simulink model "control"  (R2023a)
settings: Solver=ode45  StartTime=0.0  StopTime=T  RelTol=1e-3
values from neighbouring files (symbols this model uses):
  z = ismembertol(env.V,[X(x,x),Y(y,y)], 'ByRows', true)    [Environment.m]
undefined symbols (not defined in the file or in its folder): hctrl, Tc
settings Model: Creator=Luca  LastModifiedBy=nick
settings SolverCC: AlgebraicLoopSolver=TrustRegion
settings DataIOCC: ReturnWorkspaceOutputs=off
settings DebuggingCC: UnconnectedInputMsg=warning  UnconnectedOutputMsg=warning  UnconnectedLineMsg=warning  ArithmeticOperatorsInVariantConditions=warning
settings ModelReferenceCC: EnableRefExpFcnMdlSchedulingChecks=on
settings SFSimCC: CustomCodeUndefinedFunction=UseInterfaceOnly

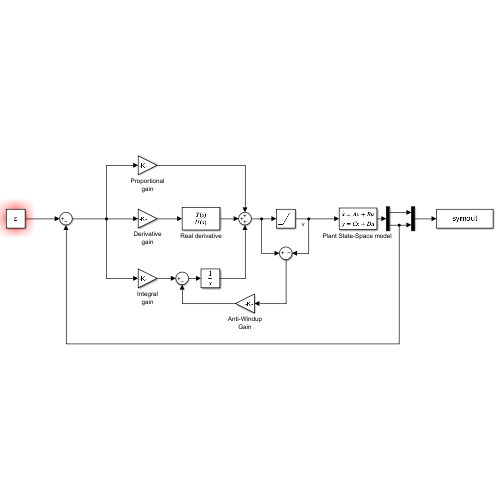
[thumbnail: Simulink's stored preview of the top-level diagram]
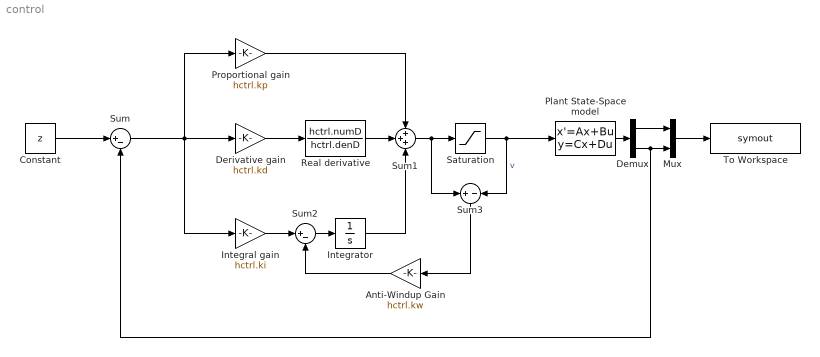
== system control ==
  Anti-Windup Gain : Gain  Gain=hctrl.kw
  Constant : Constant  Value=z  SampleTime=Tc
  Demux : Demux  Outputs=2
  Derivative gain : Gain  Gain=hctrl.kd
  Integral gain : Gain  Gain=hctrl.ki
  Integrator : Integrator
  Mux : Mux  Inputs=2
  "Plant State-Space model " : StateSpace  A=hctrl.A  B=hctrl.B  C=hctrl.C  D=hctrl.D  InitialCondition=[hctrl.vh0; hctrl.h0]
  Proportional gain : Gain  Gain=hctrl.kp
  Real derivative : TransferFcn  Numerator=hctrl.numD  Denominator=hctrl.denD
  Saturation : Saturate  UpperLimit=5  LowerLimit=-3
  Sum : Sum  Inputs=|+-
  Sum1 : Sum  Inputs=+++
  Sum2 : Sum  Inputs=|+-
  Sum3 : Sum  Inputs=+-
  To Workspace : ToWorkspace  VariableName=symout  SaveFormat=Timeseries  SampleTime=Tc
  wires:
  Constant/1 -> Sum/1
  Sum2/1 -> Integrator/1
  Saturation/1 -> "Plant State-Space model "/1, Sum3/2  "v"
  Integral gain/1 -> Sum2/1
  Sum1/1 -> Sum3/1, Saturation/1
  Anti-Windup Gain/1 -> Sum2/2
  Integrator/1 -> Sum1/3
  Real derivative/1 -> Sum1/2
  Proportional gain/1 -> Sum1/1
  Derivative gain/1 -> Real derivative/1
  Sum3/1 -> Anti-Windup Gain/1
  Sum/1 -> Derivative gain/1, Integral gain/1, Proportional gain/1
  "Plant State-Space model "/1 -> Demux/1
  Demux/2 -> Mux/2, Sum/2
  Demux/1 -> Mux/1
  Mux/1 -> To Workspace/1
